simulink model "Examen10Julio"  (R2022b)
settings: Solver=VariableStepAuto  StartTime=0.0  StopTime=10.0  RelTol=1e-3
values from neighbouring files (symbols this model uses):
  A = [-1 -2 ... (first row only)    [ABinvariantes11deJunio.m]    (also in Convertibility.m = [0 1 0  0 0; DivirsoresElementales.m = [1 0 -1; 0 1 0; 0 0 2]; Examen.m = [1 1;0 1]; Examen2.m = [0 0  0 0 0)
  B = [1 ... (first row only)    [ABinvariantes11deJunio.m]    (also in Convertibility.m = [0 0; Examen.m = [1;0]; Examen2.m = [1 0; Sestrella.m = [0;1;0])
  D = [2 -3]    [ABinvariantes11deJunio.m]    (also in Examen2.m = [0 0 0 1 0]; V_estrella.m = [0 0 0 1 0]; Westrella.m = [1 0)
settings Model: Creator=raul  LastModifiedBy=raul

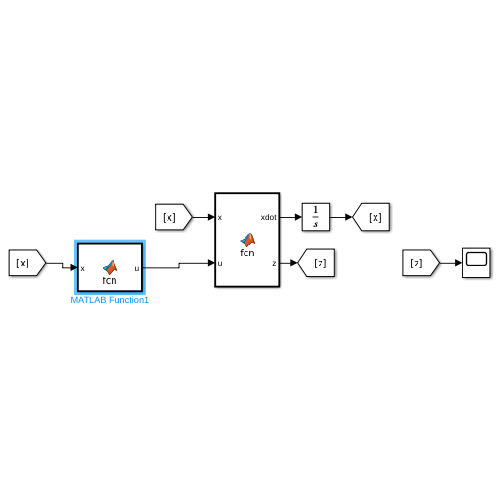
[thumbnail: Simulink's stored preview of the top-level diagram]
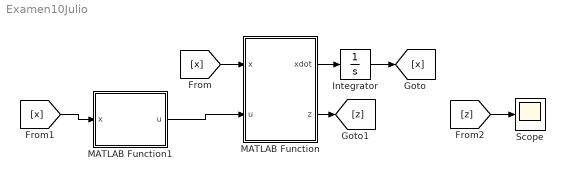
== system Examen10Julio ==
  Integrator : Integrator  InitialCondition=[1; 1; 1; 1; 1]
  MATLAB Function : MATLAB Function  TreatAsAtomicUnit=on
  MATLAB Function1 : MATLAB Function  TreatAsAtomicUnit=on
  Scope : Scope
  wires:
  MATLAB Function/1(xdot) -> Integrator/1
  Integrator/1 -> [x]
  [x] -> MATLAB Function/1(x)
  MATLAB Function/2(z) -> [z]
  MATLAB Function1/1(u) -> MATLAB Function/2(u)
  [z] -> Scope/1
  [x] -> MATLAB Function1/1(x)

== matlab function Examen10Julio/MATLAB Function1 ==
  data: u output; x input
function u = fcn(x)

F=[ 3.9866   -0.0000  -13.4243   -9.5273   -1.4755;
   -0.0241    0.0000   30.1820   31.1162   10.0134];
u=-F*x;

== matlab function Examen10Julio/MATLAB Function ==
  data: xdot output; x input; u input; z output; A parameter; B parameter; D parameter
function [xdot,z] = fcn(x,u,A, B, D)

xdot=A*x+B*u;

z=D*x;
